simulink model "Converter3"  (R2022b)
settings: Solver=VariableStepAuto  StartTime=0.0  StopTime=0.5  RelTol=1e-3
libraries: spsCurrentMeasurementLib x7, spsVoltageMeasurementLib x7, spsSeriesRLCBranchLib x6, spsDiodeLib x3, spsMosfetLib x2, spsDCVoltageSourceLib x1, spspowerguiLib x1
settings Model: Creator=91637  LastModifiedBy=User
settings SolverCC: AlgebraicLoopSolver=TrustRegion
settings DebuggingCC: SFMachineParentedDataDiag=warning
settings RTWCC: DLArmComputeVersion=19.05

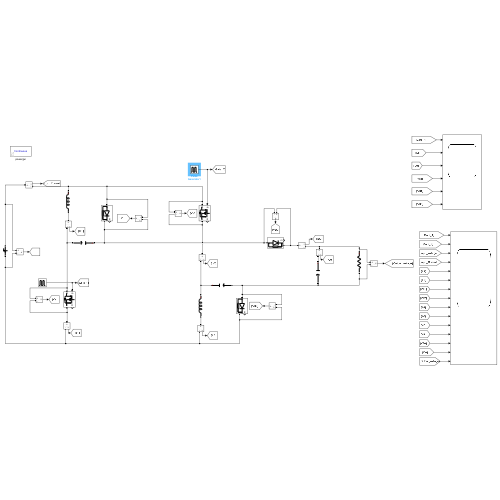
[thumbnail: Simulink's stored preview of the top-level diagram]
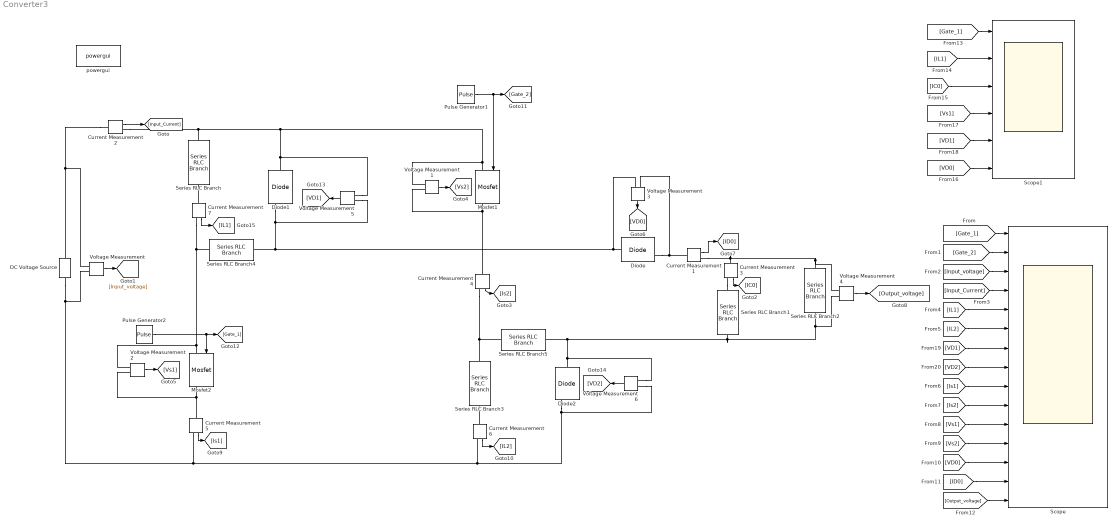
== system Converter3 ==
  Current Measurement{1..7} (7 alike) : spsCurrentMeasurementLib/Current Measurement  PhasorSimulation=off  OutputType=Complex  PSBequivalent=0
  DC Voltage Source : spsDCVoltageSourceLib/DC Voltage Source  Amplitude=12  Measurements=None
  Diode : spsDiodeLib/Diode  Ron=0.001  Lon=0  Vf=0.8  IC=0  UseSnubber=0  Rs=500  Cs=250e-9  Measurements=on
  Diode1 : spsDiodeLib/Diode  Ron=0.001  Lon=0  Vf=0.8  IC=0  UseSnubber=0  Rs=500  Cs=250e-9  Measurements=on
  Diode2 : spsDiodeLib/Diode  Ron=0.001  Lon=0  Vf=0.8  IC=0  UseSnubber=0  Rs=500  Cs=250e-9  Measurements=on
  Mosfet1 : spsMosfetLib/Mosfet  Ron=0.1  Lon=0  Rd=0.01  Vfd=0  IC=0  Rs=1e5  Cs=inf  Measurements=on
  Mosfet2 : spsMosfetLib/Mosfet  Ron=0.1  Lon=0  Rd=0.01  Vfd=0  IC=0  Rs=1e5  Cs=inf  Measurements=on
  Pulse Generator1 : DiscretePulseGenerator  PulseType=Time based  Amplitude=5  Period=1/100000  PulseWidth=73
  Pulse Generator2 : DiscretePulseGenerator  PulseType=Time based  Amplitude=5  Period=1/100000  PulseWidth=73
  Scope : Scope  NumInputPorts=15
  Scope1 : Scope  NumInputPorts=6
  Series RLC Branch : spsSeriesRLCBranchLib/Series RLC Branch  LConnTagsString=__new0  RConnTagsString=__new0  BranchType=L  Resistance=1  Inductance=92.64e-6  SetiL0=off  InitialCurrent=0  Capacitance=1e-6  Setx0=off  InitialVoltage=0  Measurements=None
  Series RLC Branch1 : spsSeriesRLCBranchLib/Series RLC Branch  LConnTagsString=__new0  RConnTagsString=__new0  BranchType=C  Resistance=1  Inductance=1e-3  SetiL0=off  InitialCurrent=0  Capacitance=22e-6  Setx0=off  InitialVoltage=0  Measurements=None
  Series RLC Branch2 : spsSeriesRLCBranchLib/Series RLC Branch  LConnTagsString=__new0  RConnTagsString=__new0  BranchType=R  Resistance=90  Inductance=1e-3  SetiL0=off  InitialCurrent=0  Capacitance=1e-6  Setx0=off  InitialVoltage=0  Measurements=None
  Series RLC Branch3 : spsSeriesRLCBranchLib/Series RLC Branch  LConnTagsString=__new0  RConnTagsString=__new0  BranchType=L  Resistance=1  Inductance=92.64e-6  SetiL0=off  InitialCurrent=0  Capacitance=1e-6  Setx0=off  InitialVoltage=0  Measurements=None
  Series RLC Branch4 : spsSeriesRLCBranchLib/Series RLC Branch  LConnTagsString=__new0  RConnTagsString=__new0  BranchType=C  Resistance=1  Inductance=1e-3  SetiL0=off  InitialCurrent=0  Capacitance=74e-6  Setx0=off  InitialVoltage=0  Measurements=None
  Series RLC Branch5 : spsSeriesRLCBranchLib/Series RLC Branch  LConnTagsString=__new0  RConnTagsString=__new0  BranchType=C  Resistance=1  Inductance=1e-3  SetiL0=off  InitialCurrent=0  Capacitance=74e-6  Setx0=off  InitialVoltage=0  Measurements=None
  Voltage Measurement{,1..6} (7 alike) : spsVoltageMeasurementLib/Voltage Measurement  PhasorSimulation=off  OutputType=Complex  PSBequivalent=0
  powergui : spspowerguiLib/powergui  Priority=1  SimulationMode=Continuous  SampleTime=50e-6  frequency=60  Iterations=50  frequencyindice=0  Pbase=100e6  ErrMax=1e-4  UnitsV=kV  UnitsW=MW  buscounter=0  FunctionMessages=off  echomessages=off  EnableUseOfTLC=off  CurrentSourceSwitches=off  DisableSnubberDevices=off  DisableRonSwitches=off  DisableVfSwitches=off  DisplayEquations=off  AutomaticDiscreteSolvers=off  SolverType=Tustin/Backward Euler (TBE)  Interpol=off  ExternalGateDelay=off  methode=off  Ts=100  x0status=blocks  SPID=on  SwTol=0  HookPort=off  NonlinearTolerance=1e-4  nMaxIteration=100  ContinueOnMaxIteration=off  RestoreLinks=warning  ResistiveCurrentMeasurement=off  Frange=[0:2:500]  Ylog=off  Xlog=on  ShowGrid=off  save=off  variable=ZData  structure=0  ZoomFFT=off  StartTime=0.0  cycles=1  DisplayStyle=1  fundamental=60  FreqAxis=off  MaxFrequency=1000  frequencyindicesteady=1  RmsSteady=1  display=off
  wires:
  Voltage Measurement5/1 -> [VD1]
  Pulse Generator1/1 -> Mosfet1/1, [Gate_2]
  Pulse Generator2/1 -> Mosfet2/1, [Gate_1]
  Current Measurement1/1 -> [ID0]
  Voltage Measurement1/1 -> [Vs2]
  Voltage Measurement4/1 -> [Output_voltage]
  Voltage Measurement/1 -> [Input_voltage]
  Voltage Measurement3/1 -> [VD0]
  Current Measurement4/1 -> [Is2]
  Current Measurement6/1 -> [IL2]
  Voltage Measurement2/1 -> [Vs1]
  Current Measurement2/1 -> [Input_Current]
  Current Measurement5/1 -> [Is1]
  Voltage Measurement6/1 -> [VD2]
  Current Measurement7/1 -> [IL1]
  Current Measurement3/1 -> [IC0]
  [IC0] -> Scope1/3
  [VD0] -> Scope1/6
  [VD1] -> Scope1/5
  [Vs1] -> Scope1/4
  [IL1] -> Scope1/2
  [Gate_1] -> Scope1/1
  [VD1] -> Scope/7
  [Is1] -> Scope/9
  [ID0] -> Scope/14
  [Is2] -> Scope/10
  [Output_voltage] -> Scope/15
  [Gate_1] -> Scope/1
  [Gate_2] -> Scope/2
  [Input_Current] -> Scope/4
  [IL1] -> Scope/5
  [Vs1] -> Scope/11
  [Vs2] -> Scope/12
  [IL2] -> Scope/6
  [Input_voltage] -> Scope/3
  [VD0] -> Scope/13
  [VD2] -> Scope/8
  connections:
  Diode1/RConn1 -- Voltage Measurement5/LConn1 -- Voltage Measurement3/LConn2 -- Diode/LConn1 -- Series RLC Branch4/LConn1
  DC Voltage Source/LConn1 -- Voltage Measurement/LConn2 -- Current Measurement5/RConn1 -- Voltage Measurement6/LConn1 -- Diode2/RConn1 -- Current Measurement6/RConn1
  Current Measurement1/RConn1 -- Current Measurement3/LConn1 -- Voltage Measurement4/LConn1 -- Series RLC Branch2/LConn1
  Voltage Measurement4/LConn2 -- Voltage Measurement6/LConn2 -- Diode2/LConn1 -- Series RLC Branch5/RConn1 -- Series RLC Branch1/RConn1 -- Series RLC Branch2/RConn1
  Current Measurement2/RConn1 -- Voltage Measurement1/LConn1 -- Mosfet1/LConn1 -- Diode1/LConn1 -- Voltage Measurement5/LConn2 -- Series RLC Branch/LConn1
  Diode/RConn1 -- Voltage Measurement3/LConn1 -- Current Measurement1/LConn1
  Current Measurement4/LConn1 -- Voltage Measurement1/LConn2 -- Mosfet1/RConn1
  Mosfet2/LConn1 -- Current Measurement7/RConn1 -- Series RLC Branch4/RConn1 -- Voltage Measurement2/LConn1
  Current Measurement2/LConn1 -- DC Voltage Source/RConn1 -- Voltage Measurement/LConn1
  Current Measurement5/LConn1 -- Voltage Measurement2/LConn2 -- Mosfet2/RConn1
  Current Measurement6/LConn1 -- Series RLC Branch3/RConn1
  Current Measurement4/RConn1 -- Series RLC Branch5/LConn1 -- Series RLC Branch3/LConn1
  Current Measurement7/LConn1 -- Series RLC Branch/RConn1
  Current Measurement3/RConn1 -- Series RLC Branch1/LConn1
